simulink model "QCS_Sim_miu"  (R2023b)
settings: Solver=ode45  StartTime=0.0  StopTime=4  RelTol=1e-3  EnableMultiTasking=on
libraries: cstblocks x9, RCTblocks x1
settings Model: Creator=Mokrane  LastModifiedBy=haoyuan
settings SolverCC: AlgebraicLoopSolver=TrustRegion
settings DataIOCC: LimitDataPoints=on  SaveFormat=Array  SignalLoggingSaveFormat=ModelDataLogs  ReturnWorkspaceOutputs=off  SignalLoggingName=sigsOut
settings DebuggingCC: SaveWithParameterizedLinksMsg=none  UnderspecifiedInitializationDetection=Classic  MergeDetectMultiDrivingBlocksExec=none  SignalResolutionControl=TryResolveAllWithWarning  MultiTaskDSMMsg=warning  MultiTaskCondExecSysMsg=none  UnconnectedInputMsg=warning  UnconnectedOutputMsg=warning  UnconnectedLineMsg=warning  ArithmeticOperatorsInVariantConditions=warning
settings HardwareCC: ProdBitPerPointer=32  ProdBitPerSizeT=32  ProdBitPerPtrDiffT=32  ProdLargestAtomicFloat=None  ProdIntDivRoundTo=Undefined  ProdEndianess=Unspecified  ProdWordSize=32  ProdHWDeviceType=32-bit Generic  TargetUnknown=on
settings ModelReferenceCC: EnableRefExpFcnMdlSchedulingChecks=on  PropagateSignalLabelsOutOfModel=off
settings SFSimCC: SimUseLocalCustomCode=off  CustomCodeUndefinedFunction=UseInterfaceOnly
settings RTWCC: RTWUseLocalCustomCode=off
settings GRTTargetCC: TargetLangStandard=C89/C90 (ANSI)  CombineOutputUpdateFcns=off  GRTInterface=on
settings ConfigComp: CovMetricSettings=dw  CovSaveCumulativeToWorkspaceVar=on  CovSaveSingleToWorkspaceVar=on  CovExternalEMLEnable=off

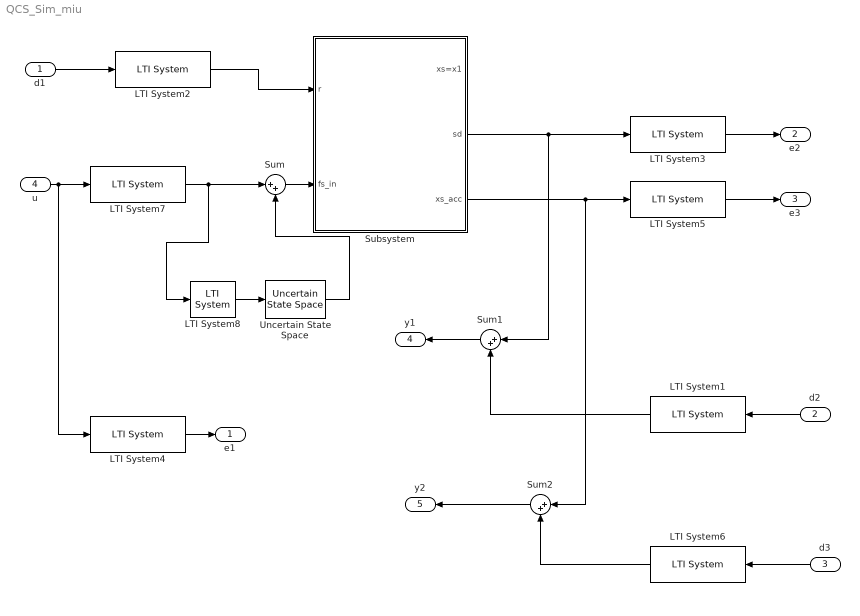
== system QCS_Sim_miu ==
  d1 : Inport
  d2 : Inport  Port=2
  d3 : Inport  Port=3
  u : Inport  Port=4
  LTI System1 : cstblocks/LTI System  sys=Wd2  IC=[]  PadeOrder=0
  LTI System2 : cstblocks/LTI System  sys=Wroad  IC=[]  PadeOrder=0
  LTI System3 : cstblocks/LTI System  sys=Wsd  IC=[]  PadeOrder=0
  LTI System4 : cstblocks/LTI System  sys=Wact  IC=[]  PadeOrder=0
  LTI System5 : cstblocks/LTI System  sys=Wab  IC=[]  PadeOrder=0
  LTI System6 : cstblocks/LTI System  sys=Wd3  IC=[]  PadeOrder=0
  LTI System7 : cstblocks/LTI System  sys=Act  IC=[]  PadeOrder=0
  LTI System8 : cstblocks/LTI System  sys=Wunc  IC=[]  PadeOrder=0
  Subsystem : Subsystem
  Sum : Sum  Inputs=|++
  Sum1 : Sum  Inputs=|++  SaturateOnIntegerOverflow=on
  Sum2 : Sum  Inputs=|++  SaturateOnIntegerOverflow=on
  Uncertain State Space : RCTblocks/Uncertain State Space  Tag=USS  USystem=unc  UValue=[]  X0=[]  uX0=[]
  e1 : Outport  VectorParamsAs1DForOutWhenUnconnected=off
  e2 : Outport  Port=2  VectorParamsAs1DForOutWhenUnconnected=off
  e3 : Outport  Port=3  VectorParamsAs1DForOutWhenUnconnected=off
  y1 : Outport  Port=4  VectorParamsAs1DForOutWhenUnconnected=off
  y2 : Outport  Port=5  VectorParamsAs1DForOutWhenUnconnected=off
  wires:
  d1/1 -> LTI System2/1
  LTI System2/1 -> Subsystem/1(r)
  LTI System4/1 -> e1/1
  Subsystem/2(sd) -> LTI System3/1, Sum1/1
  LTI System3/1 -> e2/1
  Subsystem/3(xs_acc) -> Sum2/1, LTI System5/1
  LTI System5/1 -> e3/1
  d2/1 -> LTI System1/1
  d3/1 -> LTI System6/1
  LTI System1/1 -> Sum1/2
  Sum1/1 -> y1/1
  LTI System6/1 -> Sum2/2
  Sum2/1 -> y2/1
  u/1 -> LTI System7/1, LTI System4/1
  LTI System7/1 -> Sum/1, LTI System8/1
  LTI System8/1 -> Uncertain State Space/1
  Sum/1 -> Subsystem/2(fs_in)
  Uncertain State Space/1 -> Sum/2

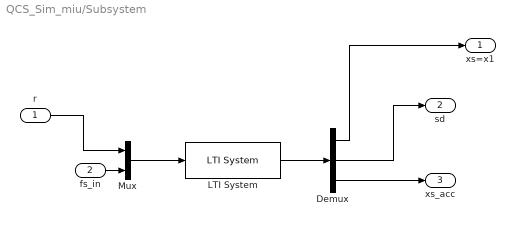
== system QCS_Sim_miu/Subsystem ==
  r : Inport
  fs_in : Inport  Port=2
  Demux : Demux  Outputs=3
  LTI System : cstblocks/LTI System  sys=qcar  IC=[]  PadeOrder=0
  Mux : Mux  Inputs=2
  xs=x1 : Outport  VectorParamsAs1DForOutWhenUnconnected=off
  sd : Outport  Port=2  VectorParamsAs1DForOutWhenUnconnected=off
  xs_acc : Outport  Port=3  VectorParamsAs1DForOutWhenUnconnected=off
  wires:
  Demux/2 -> sd/1
  Demux/3 -> xs_acc/1
  Demux/1 -> xs=x1/1
  r/1 -> Mux/1
  fs_in/1 -> Mux/2
  Mux/1 -> LTI System/1
  LTI System/1 -> Demux/1
